simulink model "untitled"  (R2015a)
settings: Solver=ode45  StartTime=0.0  StopTime=10.0  RelTol=1e-3
libraries: powerlib x38
settings Model: CovSFcnEnable=off  Creator=SELVA  LastModifiedBy=SELVA SAM
settings DebuggingCC: SolverPrmCheckMsg=warning

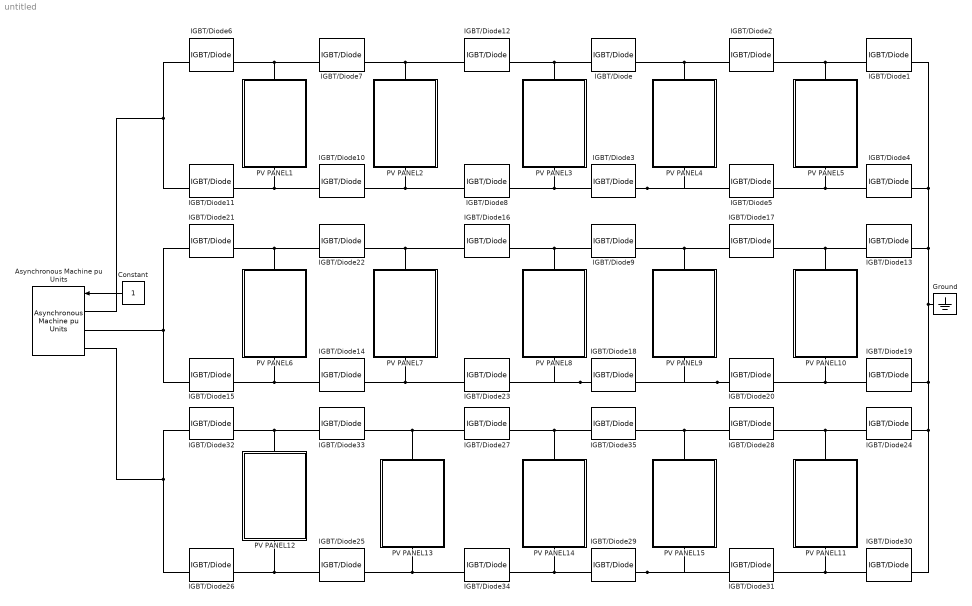
== system untitled ==
  Asynchronous Machine pu Units : powerlib/Machines/Asynchronous Machine pu Units  RotorType=Squirrel-cage  PresetModel=No  MechanicalLoad=Torque Tm  ShowDetailedParameters=on  ReferenceFrame=Rotor  Units=pu  MeasurementBus=off  NominalParameters=[3730 460 60]  Stator=[0.01965 0.0397]  Rotor=[0.01909 0.0397]  Cage1=[0.01909 0.0397]  Cage2=[0.01909 0.0397]  Lm=1.354  Mechanical=[0.09526 0.05479 2]  PolePairs=2  InitialConditions="[ 1,0   0,0,0   0,0,0 ]"  SimulateSaturation=off  Saturation="[0.212,0.4201,0.8125,1.0979,1.4799,2.2457,3.2586,4.5763,6.4763 ;   0.5,0.7,0.9,1,1.1,1.2 ,1.3,1.4,1.5]"  LoadFlowParameters=0  TsPowergui=0  TsBlock=-1  IterativeModel=Trapezoidal non iterative  Pmec=0
  Constant : Constant
  Ground : powerlib/Elements/Ground  LConnTagsString=a
  IGBT/Diode{,1..35} (36 alike) : powerlib/Power Electronics/IGBT//Diode  Ron=1e-3  Rs=1e5  Cs=inf  Measurements=on
  PV PANEL1 : Subsystem
      mask Display: image('C:\Users\SELVA SAM\Downloads\2.jpg')
  PV PANEL10 : Subsystem
      mask Display: image('C:\Users\SELVA SAM\Downloads\2.jpg')
  PV PANEL11 : Subsystem
      mask Display: image('C:\Users\SELVA SAM\Downloads\2.jpg')
  PV PANEL12 : Subsystem
      mask Display: image('C:\Users\SELVA SAM\Downloads\2.jpg')
  PV PANEL13 : Subsystem
      mask Display: image('C:\Users\SELVA SAM\Downloads\2.jpg')
  PV PANEL14 : Subsystem
      mask Display: image('C:\Users\SELVA SAM\Downloads\2.jpg')
  PV PANEL15 : Subsystem
      mask Display: image('C:\Users\SELVA SAM\Downloads\2.jpg')
  PV PANEL2 : Subsystem
      mask Display: image('C:\Users\SELVA SAM\Downloads\2.jpg')
  PV PANEL3 : Subsystem
      mask Display: image('C:\Users\SELVA SAM\Downloads\2.jpg')
  PV PANEL4 : Subsystem
      mask Display: image('C:\Users\SELVA SAM\Downloads\2.jpg')
  PV PANEL5 : Subsystem
      mask Display: image('C:\Users\SELVA SAM\Downloads\2.jpg')
  PV PANEL6 : Subsystem
      mask Display: image('C:\Users\SELVA SAM\Downloads\2.jpg')
  PV PANEL7 : Subsystem
      mask Display: image('C:\Users\SELVA SAM\Downloads\2.jpg')
  PV PANEL8 : Subsystem
      mask Display: image('C:\Users\SELVA SAM\Downloads\2.jpg')
  PV PANEL9 : Subsystem
      mask Display: image('C:\Users\SELVA SAM\Downloads\2.jpg')
  wires:
  Constant/1 -> Asynchronous Machine pu Units/1
  connections:
  IGBT/Diode2/RConn1 -- IGBT/Diode/RConn1 -- PV PANEL4/LConn1
  IGBT/Diode1/LConn1 -- PV PANEL5/LConn1 -- IGBT/Diode2/LConn1
  IGBT/Diode3/LConn1 -- IGBT/Diode5/LConn1 -- PV PANEL4/RConn1
  IGBT/Diode4/RConn1 -- PV PANEL5/RConn1 -- IGBT/Diode5/RConn1
  IGBT/Diode24/RConn1 -- Ground/LConn1 -- IGBT/Diode1/RConn1 -- IGBT/Diode4/LConn1 -- IGBT/Diode13/RConn1 -- IGBT/Diode19/LConn1 -- IGBT/Diode30/LConn1
  IGBT/Diode6/LConn1 -- IGBT/Diode7/LConn1 -- PV PANEL1/LConn1
  IGBT/Diode12/RConn1 -- PV PANEL2/LConn1 -- IGBT/Diode7/RConn1
  IGBT/Diode11/RConn1 -- IGBT/Diode10/RConn1 -- PV PANEL1/RConn1
  IGBT/Diode10/LConn1 -- IGBT/Diode8/LConn1 -- PV PANEL2/RConn1
  IGBT/Diode12/LConn1 -- PV PANEL3/LConn1 -- IGBT/Diode/LConn1
  IGBT/Diode8/RConn1 -- PV PANEL3/RConn1 -- IGBT/Diode3/RConn1
  IGBT/Diode11/LConn1 -- IGBT/Diode6/RConn1 -- Asynchronous Machine pu Units/LConn1
  IGBT/Diode17/RConn1 -- IGBT/Diode9/RConn1 -- PV PANEL9/LConn1
  IGBT/Diode13/LConn1 -- IGBT/Diode17/LConn1 -- PV PANEL10/LConn1
  IGBT/Diode20/LConn1 -- IGBT/Diode18/LConn1 -- PV PANEL9/RConn1
  IGBT/Diode19/RConn1 -- PV PANEL10/RConn1 -- IGBT/Diode20/RConn1
  IGBT/Diode21/LConn1 -- PV PANEL6/LConn1 -- IGBT/Diode22/LConn1
  IGBT/Diode22/RConn1 -- PV PANEL7/LConn1 -- IGBT/Diode16/RConn1
  IGBT/Diode15/RConn1 -- PV PANEL6/RConn1 -- IGBT/Diode14/RConn1
  IGBT/Diode23/LConn1 -- IGBT/Diode14/LConn1 -- PV PANEL7/RConn1
  IGBT/Diode16/LConn1 -- PV PANEL8/LConn1 -- IGBT/Diode9/LConn1
  IGBT/Diode18/RConn1 -- IGBT/Diode23/RConn1 -- PV PANEL8/RConn1
  IGBT/Diode15/LConn1 -- IGBT/Diode21/RConn1 -- Asynchronous Machine pu Units/LConn2
  IGBT/Diode28/RConn1 -- PV PANEL15/LConn1 -- IGBT/Diode35/RConn1
  IGBT/Diode28/LConn1 -- PV PANEL11/LConn1 -- IGBT/Diode24/LConn1
  IGBT/Diode29/LConn1 -- PV PANEL15/RConn1 -- IGBT/Diode31/LConn1
  IGBT/Diode30/RConn1 -- IGBT/Diode31/RConn1 -- PV PANEL11/RConn1
  IGBT/Diode32/LConn1 -- PV PANEL12/LConn1 -- IGBT/Diode33/LConn1
  IGBT/Diode27/RConn1 -- PV PANEL13/LConn1 -- IGBT/Diode33/RConn1
  IGBT/Diode26/RConn1 -- PV PANEL12/RConn1 -- IGBT/Diode25/RConn1
  IGBT/Diode25/LConn1 -- IGBT/Diode34/LConn1 -- PV PANEL13/RConn1
  IGBT/Diode27/LConn1 -- PV PANEL14/LConn1 -- IGBT/Diode35/LConn1
  IGBT/Diode34/RConn1 -- PV PANEL14/RConn1 -- IGBT/Diode29/RConn1
  IGBT/Diode32/RConn1 -- Asynchronous Machine pu Units/LConn3 -- IGBT/Diode26/LConn1

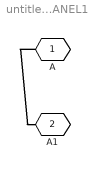
== system untitled/PV PANEL1 ==
  A : PMIOPort  Port=1  Side=Left
  A1 : PMIOPort  Port=2  Side=Right
  connections:
  A/RConn1 -- A1/RConn1

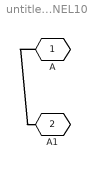
== system untitled/PV PANEL10 ==
  A : PMIOPort  Port=1  Side=Left
  A1 : PMIOPort  Port=2  Side=Right
  connections:
  A/RConn1 -- A1/RConn1

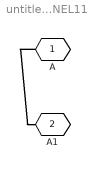
== system untitled/PV PANEL11 ==
  A : PMIOPort  Port=1  Side=Left
  A1 : PMIOPort  Port=2  Side=Right
  connections:
  A/RConn1 -- A1/RConn1

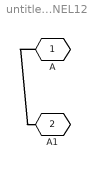
== system untitled/PV PANEL12 ==
  A : PMIOPort  Port=1  Side=Left
  A1 : PMIOPort  Port=2  Side=Right
  connections:
  A/RConn1 -- A1/RConn1

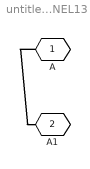
== system untitled/PV PANEL13 ==
  A : PMIOPort  Port=1  Side=Left
  A1 : PMIOPort  Port=2  Side=Right
  connections:
  A/RConn1 -- A1/RConn1

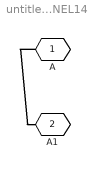
== system untitled/PV PANEL14 ==
  A : PMIOPort  Port=1  Side=Left
  A1 : PMIOPort  Port=2  Side=Right
  connections:
  A/RConn1 -- A1/RConn1

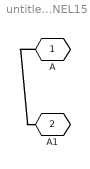
== system untitled/PV PANEL15 ==
  A : PMIOPort  Port=1  Side=Left
  A1 : PMIOPort  Port=2  Side=Right
  connections:
  A/RConn1 -- A1/RConn1

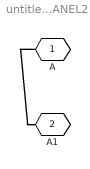
== system untitled/PV PANEL2 ==
  A : PMIOPort  Port=1  Side=Left
  A1 : PMIOPort  Port=2  Side=Right
  connections:
  A/RConn1 -- A1/RConn1

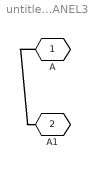
== system untitled/PV PANEL3 ==
  A : PMIOPort  Port=1  Side=Left
  A1 : PMIOPort  Port=2  Side=Right
  connections:
  A/RConn1 -- A1/RConn1

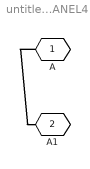
== system untitled/PV PANEL4 ==
  A : PMIOPort  Port=1  Side=Left
  A1 : PMIOPort  Port=2  Side=Right
  connections:
  A/RConn1 -- A1/RConn1

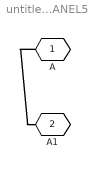
== system untitled/PV PANEL5 ==
  A : PMIOPort  Port=1  Side=Left
  A1 : PMIOPort  Port=2  Side=Right
  connections:
  A/RConn1 -- A1/RConn1

== system untitled/PV PANEL6 ==
  A : PMIOPort  Port=1  Side=Left
  A1 : PMIOPort  Port=2  Side=Right
  connections:
  A/RConn1 -- A1/RConn1

== system untitled/PV PANEL7 ==
  A : PMIOPort  Port=1  Side=Left
  A1 : PMIOPort  Port=2  Side=Right
  connections:
  A/RConn1 -- A1/RConn1

== system untitled/PV PANEL8 ==
  A : PMIOPort  Port=1  Side=Left
  A1 : PMIOPort  Port=2  Side=Right
  connections:
  A/RConn1 -- A1/RConn1

== system untitled/PV PANEL9 ==
  A : PMIOPort  Port=1  Side=Left
  A1 : PMIOPort  Port=2  Side=Right
  connections:
  A/RConn1 -- A1/RConn1
